simulink model "CHE360_Hw7_Q4"  (R2018a)
settings: Solver=VariableStepAuto  StartTime=0.0  StopTime=100000  RelTol=1e-3
settings Model: Creator=kr27867  LastModifiedBy=kr27867

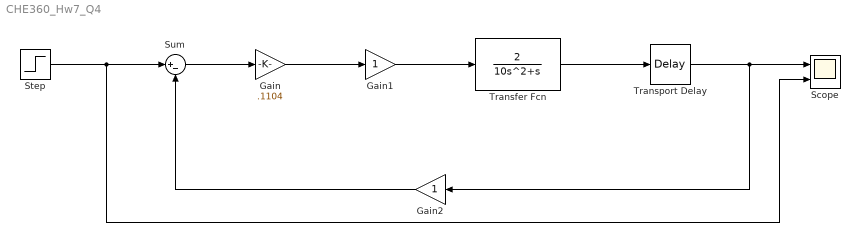
== system CHE360_Hw7_Q4 ==
  Gain : Gain  Gain=.1104
  Gain1 : Gain
  Gain2 : Gain
  Scope : Scope  NumInputPorts=2
  Step : Step  SampleTime=0
  Sum : Sum  Inputs=|+-
  Transfer Fcn : TransferFcn  Numerator=[2]  Denominator=[10 1 0]
  Transport Delay : TransportDelay  DelayTime=5
  wires:
  Step/1 -> Scope/2, Sum/1
  Sum/1 -> Gain/1
  Gain/1 -> Gain1/1
  Gain1/1 -> Transfer Fcn/1
  Gain2/1 -> Sum/2
  Transfer Fcn/1 -> Transport Delay/1
  Transport Delay/1 -> Scope/1, Gain2/1
